simulink library "ddm"  (R2021b)
settings: Solver=VariableStepAuto  StartTime=0.0  StopTime=10.0  RelTol=1e-3
undefined symbols (not defined in the file or in its folder): ADDM_FrTMTqDev_X_Nm, ADDM_RrTMTqDev_X_Nm, ENUM_ADASACCSTA_ERROR, ENUM_ADASACCSTA_OFF, ENUM_ADASACCSTA_STANDBY, ENUM_ALLOWMOV_ALLOWREADY, ENUM_APS, ENUM_BRKSTA_ERROR, ENUM_BRKSTA_OFF, ENUM_BRKSTA_ON, ENUM_BRKSW_INVALID, ENUM_BRKSW_OFF, ENUM_BRKSW_ON, ENUM_CHGPREACTERRSTA_OBCPRE, ENUM_DCDCFAULTSTA_ANYFAULTLV1, ENUM_DCDCFAULTSTA_ANYFAULTLV2, ENUM_DRIVETRAIN_AWD, ENUM_DRIVETRAIN_FWD, ENUM_DRIVETRAIN_RWD, ENUM_EDUDRTSTA_NORMAL, ENUM_EPBSTA_APPLIED, ENUM_EPBSTA_RELEASED, ENUM_ESCAPSSta_APSUNAVAILABLE, ENUM_GEARACTUALPOSN_INVALID, ENUM_GEARACTUALPOSN_P, ENUM_HVBATTREADYPRE_READY, ENUM_MCUWARN_LV0, ENUM_MCUWARN_LV1, ENUM_MCUWARN_LV2, ENUM_MCUWARN_LV3, ENUM_MCUWARN_NOERROR, ENUM_OBCFAULTSTA_ANYFAULT, ENUM_PAS_R2F2, ENUM_PDFAULT_BATTPDFAIL, ENUM_PDFAULT_DCDCDISABLE, ENUM_PDFAULT_MCUDISABLE, ENUM_PDFAULT_MCUDISCHRG, ENUM_POWERSTA_OFF, ENUM_POWERSTA_ON, ENUM_POWERSTA_READY, ENUM_POWERSTA_STANDBY, ENUM_PRESSINDI_LOW, ENUM_PUFAULT_BATTUPFAIL, ENUM_PUFAULT_DCDCENABLEFAIL, ENUM_PUFAULT_PRECHRGCHKFAIL, ENUM_PUFAULT_SAFETYCHKFAIL, ENUM_PUSTATE_COMPLETED, ENUM_PWRSTASW_OFF, ENUM_PWRSTASW_OFFA, ENUM_PWRSTASW_OFFCHVCHRG, ENUM_PWRSTASW_OFFCLVCHRG, ENUM_PWRSTASW_ON, ENUM_PWRSTASW_ONHVCHRG, ENUM_PWRSTASW_READY, ENUM_PWRSTASW_STANDBY, ENUM_RAPSErrWarnSta_NORMAL, ENUM_RAPSErrWarnSta_RAPSERRLV1, ENUM_SHIFTCOMMAND_P, ENUM_SHIFTERERRSTA_PBUTTONFAILURE, ENUM_VEHMALFUNLV_2ND ... (+463)
libraries: hcu_lib x529, $bdroot x5, simulink x4
(part 19 of 25)

== system ddm/DDM/DDM/PMM/Fault level/Fault level 2 subsystem error ==
  note: Test Pass Criteria
  note: Release Condition After Failure Decision
  note: Diagnostics and Fault Handling
  note: Test Detection Criteria
  task_time_s : Inport
  VPMM_PowerSta_enum : Inport  Port=2
  VPMM_PwrStaSW_enum : Inport  Port=3
  VDDM_C3BMS6LCCFS_flg : Inport  Port=4
  VDDM_C3CCU2LCCFS_flg : Inport  Port=5
  VDDM_MCUNF1NoComCFS_flg : Inport  Port=6
  VDDM_MCUNR1NoComCFS_flg : Inport  Port=7
  VINP_BMSWarn4_flg : Inport  Port=8
  VINP_BMSWarn5_flg : Inport  Port=9
  VINP_DCDCFaultSta_enum : Inport  Port=10
  VINP_MCUWarnFNidec_enum : Inport  Port=11
  VINP_MCUWarnRNidec_enum : Inport  Port=12
  VPMM_DrivetrainSelect_enum : Inport  Port=13
  DTC_clear_request : Inport  Port=14
  No_CAN3_BUS_OFF : Inport  Port=15
  VDDM_C3CCU2RCCFS_flg : Inport  Port=16
  VDDM_C3CCU2CSCFS_flg : Inport  Port=17
  VDDM_MCUNR1RCErrCFS_flg : Inport  Port=18
  VDDM_MCUNR1CSErrCFS_flg : Inport  Port=19
  VDDM_MCUNF1RCErrCFS_flg : Inport  Port=20
  VDDM_MCUNF1CSErrCFS_flg : Inport  Port=21
  VDDM_C3BMS6RCCFS_flg : Inport  Port=22
  VDDM_C3BMS6CSCFS_flg : Inport  Port=23
  ZoneDrMalfunLevel_enum : Inport  Port=24
  No_CAN4_BUS_OFF : Inport  Port=25
  VDDM_DrVCUNoComCFS_flg : Inport  Port=26
  ZoneFrMalfunLevel_enum : Inport  Port=27
  VDDM_FrVCUNoComCFS_flg : Inport  Port=28
  AND1 : Logic  Inputs=5  AllPortsSameDT=off  OutDataTypeStr=boolean
  AND2 : Logic  Inputs=5  AllPortsSameDT=off  OutDataTypeStr=boolean
  AND5 : Logic  Inputs=3  AllPortsSameDT=off  OutDataTypeStr=boolean
  AND6 : Logic  Inputs=3  AllPortsSameDT=off  OutDataTypeStr=boolean
  Constant1 : Constant  Value=ENUM_PWRSTASW_OFF
  Constant14 : Constant  Value=ZERO_INT
  Constant15 : Constant  Value=KDDM_FaultLvDiagnosisOffSW_flg
  Constant16 : Constant  Value=ENUM_MCUWARN_LV1
  Constant17 : Constant  Value=ENUM_DRIVETRAIN_AWD
  Constant18 : Constant  Value=ENUM_DRIVETRAIN_AWD
  Constant19 : Constant  Value=KDDM_Lv2ErrPassTO_s
  Constant2 : Constant  Value=TRUE
  Constant20 : Constant  Value=ENUM_DRIVETRAIN_FWD
  Constant21 : Constant  Value=ENUM_DRIVETRAIN_RWD
  Constant22 : Constant  Value=ENUM_MCUWARN_LV2
  Constant23 : Constant  Value=ENUM_POWERSTA_OFF
  Constant24 : Constant  Value=TRUE
  Constant25 : Constant  Value=FALSE
  Constant26 : Constant  Value=ENUM_PWRSTASW_OFF
  Constant27 : Constant  Value=FALSE
  Constant28 : Constant  Value=ENUM_MCUWARN_LV1
  Constant3 : Constant  Value=KDDM_Lv2ErrDetTO_s
  Constant36 : Constant  Value=ENUM_DCDCFAULTSTA_ANYFAULTLV2
  Constant4 : Constant  Value=KDDM_Lv2ErrPassTO_s
  Constant40 : Constant  Value=KDDM_Lv2ErrDTC_cnt
  Constant5 : Constant  Value=KDDM_Lv2ErrDTC_cnt
  Constant6 : Constant  Value=ENUM_ZONEMALFUNLV_2ND
  Constant7 : Constant  Value=ENUM_ZONEMALFUNLV_2ND
  Constant8 : Constant  Value=FALSE
  Constant9 : Constant  Value=ENUM_MCUWARN_LV2
  DTC_Couter : hcu_lib/Basic_Blocks/DTC_Couter
  DTC_Info : hcu_lib/Basic_Blocks/DTC_Info
  Delay : Delay  DelayLength=1
  Equal : RelationalOperator  Operator=~=  OutDataTypeStr=boolean  RndMeth=Simplest
  Equal1 : RelationalOperator  Operator=~=  OutDataTypeStr=boolean  RndMeth=Simplest
  Equal{2,4..5,8,14,22..28} (12 alike) : RelationalOperator  Operator===  OutDataTypeStr=boolean  RndMeth=Simplest
  Equal3 : RelationalOperator  OutDataTypeStr=boolean  RndMeth=Simplest
  Logical Operator1 : Logic  Inputs=6  AllPortsSameDT=off  OutDataTypeStr=boolean
  Logical Operator2 : Logic  Inputs=6  AllPortsSameDT=off  OutDataTypeStr=boolean
  Logical Operator3 : Logic  AllPortsSameDT=off  OutDataTypeStr=boolean
  Logical Operator6 : Logic  Operator=NOT  AllPortsSameDT=off  OutDataTypeStr=boolean
  Logical Operator7 : Logic  Operator=OR  AllPortsSameDT=off  OutDataTypeStr=boolean
  Logical Operator8 : Logic  Operator=OR  Inputs=4  AllPortsSameDT=off  OutDataTypeStr=boolean
  Logical Operator9 : Logic  Operator=OR  AllPortsSameDT=off  OutDataTypeStr=boolean
  NOT{,5..7,9..13,15,17..19,26,28} (15 alike) : Logic  Operator=NOT  AllPortsSameDT=off  OutDataTypeStr=boolean
  OR : Logic  Operator=OR  AllPortsSameDT=off  OutDataTypeStr=boolean
  OR1 : Logic  Operator=OR  AllPortsSameDT=off  OutDataTypeStr=boolean
  OR2 : Logic  Operator=OR  Inputs=6  AllPortsSameDT=off  OutDataTypeStr=boolean
  OR3 : Logic  Operator=OR  Inputs=6  AllPortsSameDT=off  OutDataTypeStr=boolean
  OR4 : Logic  Operator=OR  AllPortsSameDT=off  OutDataTypeStr=boolean
  Relational Operator : RelationalOperator  Operator=>  OutDataTypeStr=boolean  RndMeth=Simplest
  Switch{1,4..5,9} (4 alike) : Switch  Criteria=u2 ~= 0
  Terminator : Terminator
  Test Detection Criteria : hcu_lib/Basic_Blocks/Test Detection Criteria
  Timer1 : hcu_lib/Basic_Blocks/Timer
  VDDM_Lv2ErrCFS_flg : Outport
  VDDM_Lv2ErrDTC_raw32 : Outport  Port=2
  wires:
  Constant9/1 -> Equal5/2
  [VINP_MCUWarnRNidec_enum] -> Equal5/1
  Equal5/1 -> OR4/2
  OR4/1 -> Logical Operator2/1
  Switch9/1 -> Test Detection Criteria/1
  Constant8/1 -> Switch9/1
  [VDDM_Lv2ErrCFSRls_flg] -> Switch9/2
  [VDDM_Lv2ErrCFS_flg] -> DTC_Info/3
  DTC_Info/1 -> VDDM_Lv2ErrDTC_raw32/1  "VDDM_Lv2ErrDTC_raw32"
  [VDDM_Lv2ErrPass_flg] -> DTC_Info/2
  [VDDM_Lv2ErrDet_flg] -> DTC_Info/1
  [DTC_clear_request] -> DTC_Info/4
  [VDDM_ZoneDrFaultLv2_flg] -> OR3/5
  [VDDM_ZoneFrFaultLv2_flg] -> OR3/6
  [VDDM_DCDCFaultLv2_flg] -> OR3/1
  [VDDM_BMSFaultLv2_flg] -> OR3/4
  [VDDM_MCUF1FaultLv2_flg] -> OR3/3
  [VDDM_MCUR1FaultLv2_flg] -> OR3/2
  VDDM_FrVCUNoComCFS_flg/1 -> [VDDM_FrVCUNoComCFS_flg]
  ZoneFrMalfunLevel_enum/1 -> [ZoneFrMalfunLevel_enum]
  VDDM_DrVCUNoComCFS_flg/1 -> [VDDM_DrVCUNoComCFS_flg]
  No_CAN4_BUS_OFF/1 -> [No_CAN4_BUS_OFF]
  ZoneDrMalfunLevel_enum/1 -> [ZoneDrMalfunLevel_enum]
  [VDDM_ZoneFrFaultLv2_flg] -> OR2/6
  [VDDM_ZoneDrFaultLv2_flg] -> OR2/5
  NOT28/1 -> AND6/3
  [VDDM_FrVCUNoComCFS_flg] -> NOT28/1
  Equal2/1 -> AND5/1
  Constant6/1 -> Equal2/2
  [VDDM_DrVCUNoComCFS_flg] -> NOT26/1
  AND5/1 -> [VDDM_ZoneDrFaultLv2_flg]  "VDDM_ZoneDrFaultLv2_flg"
  [No_CAN4_BUS_OFF] -> AND6/2
  AND6/1 -> [VDDM_ZoneFrFaultLv2_flg]  "VDDM_ZoneFrFaultLv2_flg"
  [ZoneDrMalfunLevel_enum] -> Equal2/1
  NOT26/1 -> AND5/3
  Equal8/1 -> AND6/1
  Constant7/1 -> Equal8/2
  [ZoneFrMalfunLevel_enum] -> Equal8/1
  [No_CAN4_BUS_OFF] -> AND5/2
  VDDM_C3BMS6CSCFS_flg/1 -> [VDDM_C3BMS6CSCFS_flg]
  VDDM_C3BMS6RCCFS_flg/1 -> [VDDM_C3BMS6RCCFS_flg]
  VDDM_MCUNF1CSErrCFS_flg/1 -> [VDDM_MCUNF1CSErrCFS_flg]
  VDDM_MCUNF1RCErrCFS_flg/1 -> [VDDM_MCUNF1RCErrCFS_flg]
  VDDM_MCUNR1CSErrCFS_flg/1 -> [VDDM_MCUNR1CSErrCFS_flg]
  VDDM_MCUNR1RCErrCFS_flg/1 -> [VDDM_MCUNR1RCErrCFS_flg]
  VDDM_C3CCU2CSCFS_flg/1 -> [VDDM_C3CCU2CSCFS_flg]
  VDDM_C3CCU2RCCFS_flg/1 -> [VDDM_C3CCU2RCCFS_flg]
  [VDDM_Lv2ErrCFS_flg] -> VDDM_Lv2ErrCFS_flg/1
  Constant1/1 -> Equal1/2
  Constant2/1 -> Switch1/3
  [VPMM_PwrStaSW_enum] -> Equal1/1
  Equal1/1 -> Switch1/2
  OR3/1 -> Switch1/1
  OR2/1 -> Switch5/1
  [VDDM_BMSFaultLv2_flg] -> OR2/4
  [VDDM_MCUF1FaultLv2_flg] -> OR2/3
  [VDDM_MCUR1FaultLv2_flg] -> OR2/2
  [VDDM_DCDCFaultLv2_flg] -> OR2/1
  NOT19/1 -> AND2/5
  [VDDM_C3BMS6CSCFS_flg] -> NOT19/1
  [VINP_BMSWarn4_flg] -> OR1/1
  [VINP_BMSWarn5_flg] -> OR1/2
  [VDDM_C3BMS6LCCFS_flg] -> NOT17/1
  NOT18/1 -> AND2/4
  [No_CAN3_BUS_OFF] -> AND2/2
  OR1/1 -> AND2/1
  [VDDM_C3BMS6RCCFS_flg] -> NOT18/1
  AND2/1 -> [VDDM_BMSFaultLv2_flg]  "VDDM_BMSFaultLv2_flg"
  NOT17/1 -> AND2/3
  OR/1 -> Logical Operator1/1
  Equal23/1 -> OR/2
  Equal28/1 -> OR/1
  Constant28/1 -> Equal28/2
  [VINP_MCUWarnFNidec_enum] -> Equal28/1
  Constant17/1 -> Equal27/2
  Equal25/1 -> Logical Operator7/1
  [VPMM_DrivetrainSelect_enum] -> Equal24/1, Equal22/2
  Constant21/1 -> Equal25/1
  [VINP_MCUWarnRNidec_enum] -> Equal26/1
  NOT9/1 -> Logical Operator2/3
  [VINP_MCUWarnFNidec_enum] -> Equal23/1
  Equal26/1 -> OR4/1
  NOT15/1 -> Logical Operator1/3
  NOT10/1 -> Logical Operator2/4
  [VDDM_MCUNR1RCErrCFS_flg] -> NOT10/1
  Logical Operator9/1 -> Logical Operator1/6
  [VDDM_MCUNF1CSErrCFS_flg] -> NOT13/1
  NOT12/1 -> Logical Operator1/4
  NOT13/1 -> Logical Operator1/5
  [VDDM_MCUNF1RCErrCFS_flg] -> NOT12/1
  [No_CAN3_BUS_OFF] -> Logical Operator1/2
  [VDDM_MCUNR1CSErrCFS_flg] -> NOT11/1
  Equal27/1 -> Logical Operator7/2
  Logical Operator1/1 -> [VDDM_MCUF1FaultLv2_flg]  "VDDM_MCUF1FaultLv2_flg"
  [No_CAN3_BUS_OFF] -> Logical Operator2/2
  Logical Operator2/1 -> [VDDM_MCUR1FaultLv2_flg]  "VDDM_MCUR1FaultLv2_flg"
  Constant16/1 -> Equal26/2
  [VDDM_MCUNR1NoComCFS_flg] -> NOT9/1
  Equal24/1 -> Logical Operator9/2
  NOT11/1 -> Logical Operator2/5
  Logical Operator7/1 -> Logical Operator2/6
  [VPMM_DrivetrainSelect_enum] -> Equal25/2, Equal27/1
  [VDDM_MCUF1NoComCFS_flg] -> NOT15/1
  Equal22/1 -> Logical Operator9/1
  Constant22/1 -> Equal23/2
  Constant18/1 -> Equal24/2
  Constant20/1 -> Equal22/1
  AND1/1 -> [VDDM_DCDCFaultLv2_flg]  "VDDM_DCDCFaultLv2_flg"
  [No_CAN3_BUS_OFF] -> AND1/2
  Equal14/1 -> AND1/1
  NOT6/1 -> AND1/4
  [VDDM_C3CCU2RCCFS_flg] -> NOT6/1
  NOT7/1 -> AND1/5
  [VDDM_C3CCU2CSCFS_flg] -> NOT7/1
  [VDDM_C3CCU2LCCFS_flg] -> NOT5/1
  NOT5/1 -> AND1/3
  Equal/1 -> Switch5/2
  Constant15/1 -> Logical Operator8/4
  [VDDM_Lv2ErrCFS_flg] -> Delay/1
  Delay/1 -> NOT/1
  NOT/1 -> Logical Operator3/2
  [VDDM_Lv2ErrPass_flg] -> Logical Operator3/1
  Logical Operator3/1 -> Logical Operator8/3
  [VDDM_Lv2ErrCFSRls_flg] -> DTC_Couter/2
  Constant14/1 -> Relational Operator/2
  Switch5/1 -> Switch9/3
  Constant3/1 -> Test Detection Criteria/4
  [task_time_s] -> Timer1/3
  No_CAN3_BUS_OFF/1 -> [No_CAN3_BUS_OFF]
  DTC_clear_request/1 -> [DTC_clear_request]
  [VPMM_PwrStaSW_enum] -> Equal/1
  [VPMM_PowerSta_enum] -> Equal4/1
  Constant4/1 -> Timer1/4
  Switch4/1 -> [VDDM_Lv2ErrCFSRls_flg]  "VDDM_Lv2ErrCFSRls_flg"
  [VINP_DCDCFaultSta_enum] -> Equal14/1
  Constant23/1 -> Equal4/2
  Constant25/1 -> Switch4/3
  Constant40/1 -> Test Detection Criteria/3
  DTC_Couter/2 -> Relational Operator/1  "VDDM_Lv2ErrDTC_cnt"
  DTC_Couter/1 -> [VDDM_Lv2ErrCFS_flg]  "VDDM_Lv2ErrCFS_flg"
  Equal4/1 -> Logical Operator8/1
  [DTC_clear_request] -> Logical Operator8/2
  Timer1/1 -> Equal3/1
  Relational Operator/1 -> Terminator/1  "VDDM_Lv2ErrDFS_flg"
  Constant19/1 -> Equal3/2
  [VDDM_Lv2ErrDet_flg] -> DTC_Couter/1
  Constant24/1 -> Switch4/1
  Switch1/1 -> Timer1/2, Logical Operator6/1
  Logical Operator8/1 -> Switch4/2
  Constant27/1 -> Switch5/3
  Constant26/1 -> Equal/2
  Constant36/1 -> Equal14/2
  Logical Operator6/1 -> Timer1/1
  [task_time_s] -> Test Detection Criteria/2
  Test Detection Criteria/1 -> [VDDM_Lv2ErrDet_flg]  "VDDM_Lv2ErrDet_flg"
  Equal3/1 -> [VDDM_Lv2ErrPass_flg]  "VDDM_Lv2ErrPass_flg"
  Constant5/1 -> DTC_Couter/3
  VDDM_C3BMS6LCCFS_flg/1 -> [VDDM_C3BMS6LCCFS_flg]
  VINP_BMSWarn4_flg/1 -> [VINP_BMSWarn4_flg]
  VINP_BMSWarn5_flg/1 -> [VINP_BMSWarn5_flg]
  task_time_s/1 -> [task_time_s]
  VPMM_PwrStaSW_enum/1 -> [VPMM_PwrStaSW_enum]
  VPMM_PowerSta_enum/1 -> [VPMM_PowerSta_enum]
  VDDM_C3CCU2LCCFS_flg/1 -> [VDDM_C3CCU2LCCFS_flg]
  VPMM_DrivetrainSelect_enum/1 -> [VPMM_DrivetrainSelect_enum]
  VINP_MCUWarnRNidec_enum/1 -> [VINP_MCUWarnRNidec_enum]
  VDDM_MCUNR1NoComCFS_flg/1 -> [VDDM_MCUNR1NoComCFS_flg]
  VDDM_MCUNF1NoComCFS_flg/1 -> [VDDM_MCUF1NoComCFS_flg]
  VINP_DCDCFaultSta_enum/1 -> [VINP_DCDCFaultSta_enum]
  VINP_MCUWarnFNidec_enum/1 -> [VINP_MCUWarnFNidec_enum]

== system ddm/DDM/DDM/PMM/Fault level/Fault level 3 subsystem error ==
  note: Release Condition After Failure Decision
  note: Diagnostics and Fault Handling
  note: Test Detection Criteria
  note: Test Pass Criteria
  task_time_s : Inport
  VPMM_PowerSta_enum : Inport  Port=2
  VPMM_PwrStaSW_enum : Inport  Port=3
  VDDM_C3BMS6LCCFS_flg : Inport  Port=4
  VDDM_MCUNF1NoComCFS_flg : Inport  Port=5
  VDDM_MCUNR1NoComCFS_flg : Inport  Port=6
  VINP_BMSWarn6_flg : Inport  Port=7
  VINP_MCUWarnFNidec_enum : Inport  Port=8
  VINP_MCUWarnRNidec_enum : Inport  Port=9
  VPMM_DrivetrainSelect_enum : Inport  Port=10
  DTC_clear_request : Inport  Port=11
  No_CAN3_BUS_OFF : Inport  Port=12
  VDDM_MCUNR1RCErrCFS_flg : Inport  Port=13
  VDDM_MCUNR1CSErrCFS_flg : Inport  Port=14
  VDDM_MCUNF1RCErrCFS_flg : Inport  Port=15
  VDDM_MCUNF1CSErrCFS_flg : Inport  Port=16
  VDDM_C3BMS6RCCFS_flg : Inport  Port=17
  VDDM_C3BMS6CSCFS_flg : Inport  Port=18
  ZoneDrMalfunLevel_enum : Inport  Port=19
  No_CAN4_BUS_OFF : Inport  Port=20
  VDDM_DrVCUNoComCFS_flg : Inport  Port=21
  ZoneFrMalfunLevel_enum : Inport  Port=22
  VDDM_FrVCUNoComCFS_flg : Inport  Port=23
  AND2 : Logic  Inputs=5  AllPortsSameDT=off  OutDataTypeStr=boolean
  AND5 : Logic  Inputs=3  AllPortsSameDT=off  OutDataTypeStr=boolean
  AND6 : Logic  Inputs=3  AllPortsSameDT=off  OutDataTypeStr=boolean
  Constant1 : Constant  Value=ENUM_PWRSTASW_OFF
  Constant10 : Constant  Value=ENUM_MCUWARN_LV3
  Constant11 : Constant  Value=ENUM_DRIVETRAIN_AWD
  Constant12 : Constant  Value=KDDM_FaultLvDiagnosisOffSW_flg
  Constant13 : Constant  Value=ENUM_DRIVETRAIN_RWD
  Constant14 : Constant  Value=ZERO_INT
  Constant15 : Constant  Value=ENUM_DRIVETRAIN_AWD
  Constant16 : Constant  Value=ENUM_DRIVETRAIN_FWD
  Constant17 : Constant  Value=ENUM_MCUWARN_LV3
  Constant18 : Constant  Value=KDDM_Lv3ErrPassTO_s
  Constant19 : Constant  Value=ENUM_POWERSTA_OFF
  Constant2 : Constant  Value=TRUE
  Constant20 : Constant  Value=ENUM_ZONEMALFUNLV_3RD
  Constant21 : Constant  Value=ENUM_ZONEMALFUNLV_3RD
  Constant22 : Constant  Value=FALSE
  Constant24 : Constant  Value=TRUE
  Constant25 : Constant  Value=FALSE
  Constant26 : Constant  Value=ENUM_PWRSTASW_OFF
  Constant27 : Constant  Value=FALSE
  Constant3 : Constant  Value=KDDM_Lv3ErrDetTO_s
  Constant4 : Constant  Value=KDDM_Lv3ErrPassTO_s
  Constant40 : Constant  Value=KDDM_Lv3ErrDTC_cnt
  Constant5 : Constant  Value=KDDM_Lv3ErrDTC_cnt
  DTC_Couter : hcu_lib/Basic_Blocks/DTC_Couter
  DTC_Info : hcu_lib/Basic_Blocks/DTC_Info
  Delay : Delay  DelayLength=1
  Equal : RelationalOperator  Operator=~=  OutDataTypeStr=boolean  RndMeth=Simplest
  Equal1 : RelationalOperator  Operator=~=  OutDataTypeStr=boolean  RndMeth=Simplest
  Equal{4,8..9,11..13,16..18} (9 alike) : RelationalOperator  Operator===  OutDataTypeStr=boolean  RndMeth=Simplest
  Equal3 : RelationalOperator  OutDataTypeStr=boolean  RndMeth=Simplest
  Logical Operator1 : Logic  Inputs=6  AllPortsSameDT=off  OutDataTypeStr=boolean
  Logical Operator2 : Logic  Operator=OR  AllPortsSameDT=off  OutDataTypeStr=boolean
  Logical Operator21 : Logic  AllPortsSameDT=off  OutDataTypeStr=boolean
  Logical Operator3 : Logic  Inputs=6  AllPortsSameDT=off  OutDataTypeStr=boolean
  Logical Operator6 : Logic  Operator=NOT  AllPortsSameDT=off  OutDataTypeStr=boolean
  Logical Operator8 : Logic  Operator=OR  Inputs=4  AllPortsSameDT=off  OutDataTypeStr=boolean
  Logical Operator9 : Logic  Operator=OR  AllPortsSameDT=off  OutDataTypeStr=boolean
  NOT{,9..13,15,17..19,26,28} (12 alike) : Logic  Operator=NOT  AllPortsSameDT=off  OutDataTypeStr=boolean
  OR : Logic  Operator=OR  Inputs=5  AllPortsSameDT=off  OutDataTypeStr=boolean
  OR1 : Logic  Operator=OR  Inputs=5  AllPortsSameDT=off  OutDataTypeStr=boolean
  Relational Operator : RelationalOperator  Operator=>  OutDataTypeStr=boolean  RndMeth=Simplest
  Switch{1,4..5,9} (4 alike) : Switch  Criteria=u2 ~= 0
  Terminator : Terminator
  Test Detection Criteria : hcu_lib/Basic_Blocks/Test Detection Criteria
  Timer1 : hcu_lib/Basic_Blocks/Timer
  VDDM_Lv3ErrCFS_flg : Outport
  VDDM_Lv3ErrDTC_raw32 : Outport  Port=2
  wires:
  Switch9/1 -> Test Detection Criteria/1
  Constant22/1 -> Switch9/1
  [VDDM_Lv3ErrCFSRls_flg] -> Switch9/2
  DTC_Info/1 -> VDDM_Lv3ErrDTC_raw32/1  "VDDM_Lv3ErrDTC_raw32"
  [VDDM_Lv3ErrCFS_flg] -> DTC_Info/3
  [VDDM_Lv3ErrPass_flg] -> DTC_Info/2
  [DTC_clear_request] -> DTC_Info/4
  [VDDM_Lv3ErrDet_flg] -> DTC_Info/1
  VDDM_FrVCUNoComCFS_flg/1 -> [VDDM_FrVCUNoComCFS_flg]
  ZoneFrMalfunLevel_enum/1 -> [ZoneFrMalfunLevel_enum]
  VDDM_DrVCUNoComCFS_flg/1 -> [VDDM_DrVCUNoComCFS_flg]
  No_CAN4_BUS_OFF/1 -> [No_CAN4_BUS_OFF]
  ZoneDrMalfunLevel_enum/1 -> [ZoneDrMalfunLevel_enum]
  VDDM_C3BMS6CSCFS_flg/1 -> [VDDM_C3BMS6CSCFS_flg]
  VDDM_C3BMS6RCCFS_flg/1 -> [VDDM_C3BMS6RCCFS_flg]
  VDDM_MCUNF1CSErrCFS_flg/1 -> [VDDM_MCUNF1CSErrCFS_flg]
  VDDM_MCUNF1RCErrCFS_flg/1 -> [VDDM_MCUNF1RCErrCFS_flg]
  VDDM_MCUNR1CSErrCFS_flg/1 -> [VDDM_MCUNR1CSErrCFS_flg]
  VDDM_MCUNR1RCErrCFS_flg/1 -> [VDDM_MCUNR1RCErrCFS_flg]
  [VDDM_Lv3ErrCFS_flg] -> VDDM_Lv3ErrCFS_flg/1
  OR1/1 -> Switch1/1
  [VDDM_ZoneFrFaultLv3_flg] -> OR1/5
  Constant2/1 -> Switch1/3
  Constant1/1 -> Equal1/2
  [VPMM_PwrStaSW_enum] -> Equal1/1
  [VDDM_ZoneDrFaultLv3_flg] -> OR1/4
  [VDDM_MCUF1FaultLv3_flg] -> OR1/2
  Equal1/1 -> Switch1/2
  [VDDM_BMSFaultLv3_flg] -> OR1/3
  [VDDM_MCUR1FaultLv3_flg] -> OR1/1
  OR/1 -> Switch5/1
  [VDDM_ZoneFrFaultLv3_flg] -> OR/5
  [VDDM_ZoneDrFaultLv3_flg] -> OR/4
  [VDDM_BMSFaultLv3_flg] -> OR/3
  [VDDM_MCUF1FaultLv3_flg] -> OR/2
  [VDDM_MCUR1FaultLv3_flg] -> OR/1
  Constant15/1 -> Equal13/2
  AND5/1 -> [VDDM_ZoneDrFaultLv3_flg]  "VDDM_ZoneDrFaultLv3_flg"
  [VDDM_C3BMS6CSCFS_flg] -> NOT19/1
  NOT19/1 -> AND2/5
  Constant21/1 -> Equal9/2
  NOT18/1 -> AND2/4
  [No_CAN4_BUS_OFF] -> AND5/2
  [ZoneFrMalfunLevel_enum] -> Equal9/1
  Equal9/1 -> AND6/1
  NOT26/1 -> AND5/3
  [ZoneDrMalfunLevel_enum] -> Equal8/1
  [VINP_BMSWarn6_flg] -> AND2/1
  [VDDM_DrVCUNoComCFS_flg] -> NOT26/1
  AND2/1 -> [VDDM_BMSFaultLv3_flg]  "VDDM_BMSFaultLv3_flg"
  NOT17/1 -> AND2/3
  Constant20/1 -> Equal8/2
  Equal8/1 -> AND5/1
  [No_CAN4_BUS_OFF] -> AND6/2
  AND6/1 -> [VDDM_ZoneFrFaultLv3_flg]  "VDDM_ZoneFrFaultLv3_flg"
  [VDDM_FrVCUNoComCFS_flg] -> NOT28/1
  NOT28/1 -> AND6/3
  [VDDM_C3BMS6RCCFS_flg] -> NOT18/1
  [No_CAN3_BUS_OFF] -> AND2/2
  [VDDM_C3BMS6LCCFS_flg] -> NOT17/1
  [VDDM_MCUNF1CSErrCFS_flg] -> NOT13/1
  Constant17/1 -> Equal12/2
  Equal13/1 -> Logical Operator9/2
  Constant16/1 -> Equal11/1
  [No_CAN3_BUS_OFF] -> Logical Operator3/2
  Logical Operator9/1 -> Logical Operator3/6
  [VDDM_MCUNF1NoComCFS_flg] -> NOT15/1
  NOT13/1 -> Logical Operator3/5
  NOT12/1 -> Logical Operator3/4
  Logical Operator3/1 -> [VDDM_MCUF1FaultLv3_flg]  "VDDM_MCUF1FaultLv3_flg"
  Equal11/1 -> Logical Operator9/1
  [VDDM_MCUNF1RCErrCFS_flg] -> NOT12/1
  [VPMM_DrivetrainSelect_enum] -> Equal13/1, Equal11/2
  [VINP_MCUWarnFNidec_enum] -> Equal12/1
  Equal12/1 -> Logical Operator3/1
  NOT15/1 -> Logical Operator3/3
  Equal17/1 -> Logical Operator1/1
  NOT9/1 -> Logical Operator1/3
  Equal18/1 -> Logical Operator2/2
  Equal16/1 -> Logical Operator2/1
  [VDDM_MCUNR1NoComCFS_flg] -> NOT9/1
  Constant11/1 -> Equal18/2
  Constant13/1 -> Equal16/1
  Constant10/1 -> Equal17/2
  [VINP_MCUWarnRNidec_enum] -> Equal17/1
  [VPMM_DrivetrainSelect_enum] -> Equal16/2, Equal18/1
  NOT10/1 -> Logical Operator1/4
  [No_CAN3_BUS_OFF] -> Logical Operator1/2
  [VDDM_MCUNR1CSErrCFS_flg] -> NOT11/1
  Logical Operator2/1 -> Logical Operator1/6
  Logical Operator1/1 -> [VDDM_MCUR1FaultLv3_flg]  "VDDM_MCUR1FaultLv3_flg"
  NOT11/1 -> Logical Operator1/5
  [VDDM_MCUNR1RCErrCFS_flg] -> NOT10/1
  Constant14/1 -> Relational Operator/2
  [VDDM_Lv3ErrCFSRls_flg] -> DTC_Couter/2
  Logical Operator21/1 -> Logical Operator8/3
  [VDDM_Lv3ErrCFS_flg] -> Delay/1
  NOT/1 -> Logical Operator21/2
  Delay/1 -> NOT/1
  Constant12/1 -> Logical Operator8/4
  [VDDM_Lv3ErrPass_flg] -> Logical Operator21/1
  Switch5/1 -> Switch9/3
  Constant3/1 -> Test Detection Criteria/4
  [task_time_s] -> Timer1/3
  No_CAN3_BUS_OFF/1 -> [No_CAN3_BUS_OFF]
  DTC_clear_request/1 -> [DTC_clear_request]
  [VPMM_PwrStaSW_enum] -> Equal/1
  [VPMM_PowerSta_enum] -> Equal4/1
  Constant4/1 -> Timer1/4
  Switch4/1 -> [VDDM_Lv3ErrCFSRls_flg]  "VDDM_Lv3ErrCFSRls_flg"
  Constant19/1 -> Equal4/2
  Constant25/1 -> Switch4/3
  Constant40/1 -> Test Detection Criteria/3
  DTC_Couter/2 -> Relational Operator/1  "VDDM_Lv3ErrDTC_cnt"
  DTC_Couter/1 -> [VDDM_Lv3ErrCFS_flg]  "VDDM_Lv3ErrCFS_flg"
  Equal4/1 -> Logical Operator8/1
  [DTC_clear_request] -> Logical Operator8/2
  Timer1/1 -> Equal3/1
  Constant26/1 -> Equal/2
  Relational Operator/1 -> Terminator/1  "VDDM_Lv3ErrDFS_flg"
  Constant18/1 -> Equal3/2
  Equal/1 -> Switch5/2
  [VDDM_Lv3ErrDet_flg] -> DTC_Couter/1
  Constant24/1 -> Switch4/1
  Switch1/1 -> Timer1/2, Logical Operator6/1
  Constant27/1 -> Switch5/3
  Logical Operator8/1 -> Switch4/2
  Logical Operator6/1 -> Timer1/1
  [task_time_s] -> Test Detection Criteria/2
  Test Detection Criteria/1 -> [VDDM_Lv3ErrDet_flg]  "VDDM_Lv3ErrDet_flg"
  Equal3/1 -> [VDDM_Lv3ErrPass_flg]  "VDDM_Lv3ErrPass_flg"
  Constant5/1 -> DTC_Couter/3
  VDDM_C3BMS6LCCFS_flg/1 -> [VDDM_C3BMS6LCCFS_flg]
  VINP_MCUWarnFNidec_enum/1 -> [VINP_MCUWarnFNidec_enum]
  VDDM_MCUNF1NoComCFS_flg/1 -> [VDDM_MCUNF1NoComCFS_flg]
  VDDM_MCUNR1NoComCFS_flg/1 -> [VDDM_MCUNR1NoComCFS_flg]
  VINP_MCUWarnRNidec_enum/1 -> [VINP_MCUWarnRNidec_enum]
  VPMM_DrivetrainSelect_enum/1 -> [VPMM_DrivetrainSelect_enum]
  VPMM_PowerSta_enum/1 -> [VPMM_PowerSta_enum]
  VPMM_PwrStaSW_enum/1 -> [VPMM_PwrStaSW_enum]
  task_time_s/1 -> [task_time_s]
  VINP_BMSWarn6_flg/1 -> [VINP_BMSWarn6_flg]

== system ddm/DDM/DDM/PMM/Fault level/Fault level 4 subsystem error1 ==
  note: Test Pass Criteria
  note: Release Condition After Failure Decision
  note: Diagnostics and Fault Handling
  note: Test Detection Criteria
  task_time_s : Inport
  VPMM_PowerSta_enum : Inport  Port=2
  VPMM_PwrStaSW_enum : Inport  Port=3
  VDDM_C3BMS6LCCFS_flg : Inport  Port=4
  VINP_BMSWarn7_flg : Inport  Port=5
  VINP_BMSWarn8_flg : Inport  Port=6
  DTC_clear_request : Inport  Port=7
  No_CAN3_BUS_OFF : Inport  Port=8
  VDDM_C3BMS6RCCFS_flg : Inport  Port=9
  VDDM_C3BMS6CSCFS_flg : Inport  Port=10
  ZoneDrMalfunLevel_enum : Inport  Port=11
  No_CAN4_BUS_OFF : Inport  Port=12
  VDDM_DrVCUNoComCFS_flg : Inport  Port=13
  ZoneFrMalfunLevel_enum : Inport  Port=14
  VDDM_FrVCUNoComCFS_flg : Inport  Port=15
  AND2 : Logic  Inputs=5  AllPortsSameDT=off  OutDataTypeStr=boolean
  AND5 : Logic  Inputs=3  AllPortsSameDT=off  OutDataTypeStr=boolean
  AND6 : Logic  Inputs=3  AllPortsSameDT=off  OutDataTypeStr=boolean
  Constant1 : Constant  Value=ENUM_PWRSTASW_OFF
  Constant12 : Constant  Value=KDDM_FaultLvDiagnosisOffSW_flg
  Constant14 : Constant  Value=ZERO_INT
  Constant18 : Constant  Value=KDDM_Lv4ErrPassTO_s
  Constant19 : Constant  Value=ENUM_POWERSTA_OFF
  Constant2 : Constant  Value=TRUE
  Constant22 : Constant  Value=FALSE
  Constant24 : Constant  Value=TRUE
  Constant25 : Constant  Value=FALSE
  Constant26 : Constant  Value=ENUM_PWRSTASW_OFF
  Constant27 : Constant  Value=FALSE
  Constant3 : Constant  Value=KDDM_Lv4ErrDetTO_s
  Constant4 : Constant  Value=KDDM_Lv4ErrPassTO_s
  Constant40 : Constant  Value=KDDM_Lv4ErrDTC_cnt
  Constant5 : Constant  Value=KDDM_Lv4ErrDTC_cnt
  Constant6 : Constant  Value=ENUM_ZONEMALFUNLV_4TH
  Constant7 : Constant  Value=ENUM_ZONEMALFUNLV_4TH
  DTC_Couter : hcu_lib/Basic_Blocks/DTC_Couter
  DTC_Info : hcu_lib/Basic_Blocks/DTC_Info
  Delay : Delay  DelayLength=1
  Equal : RelationalOperator  Operator=~=  OutDataTypeStr=boolean  RndMeth=Simplest
  Equal1 : RelationalOperator  Operator===  OutDataTypeStr=boolean  RndMeth=Simplest
  Equal2 : RelationalOperator  Operator=~=  OutDataTypeStr=boolean  RndMeth=Simplest
  Equal3 : RelationalOperator  OutDataTypeStr=boolean  RndMeth=Simplest
  Equal4 : RelationalOperator  Operator===  OutDataTypeStr=boolean  RndMeth=Simplest
  Equal8 : RelationalOperator  Operator===  OutDataTypeStr=boolean  RndMeth=Simplest
  Logical Operator21 : Logic  AllPortsSameDT=off  OutDataTypeStr=boolean
  Logical Operator6 : Logic  Operator=NOT  AllPortsSameDT=off  OutDataTypeStr=boolean
  Logical Operator8 : Logic  Operator=OR  Inputs=4  AllPortsSameDT=off  OutDataTypeStr=boolean
  NOT{,17..19,26,28} (6 alike) : Logic  Operator=NOT  AllPortsSameDT=off  OutDataTypeStr=boolean
  OR : Logic  Operator=OR  Inputs=3  AllPortsSameDT=off  OutDataTypeStr=boolean
  OR1 : Logic  Operator=OR  AllPortsSameDT=off  OutDataTypeStr=boolean
  OR2 : Logic  Operator=OR  Inputs=3  AllPortsSameDT=off  OutDataTypeStr=boolean
  Relational Operator : RelationalOperator  Operator=>  OutDataTypeStr=boolean  RndMeth=Simplest
  Switch{1,4..5,9} (4 alike) : Switch  Criteria=u2 ~= 0
  Terminator : Terminator
  Test Detection Criteria : hcu_lib/Basic_Blocks/Test Detection Criteria
  Timer1 : hcu_lib/Basic_Blocks/Timer
  VDDM_Lv4ErrCFS_flg : Outport
  VDDM_Lv4ErrDTC_raw32 : Outport  Port=2
  wires:
  Switch9/1 -> Test Detection Criteria/1
  Constant22/1 -> Switch9/1
  [VDDM_Lv4ErrCFSRls_flg] -> Switch9/2
  DTC_Info/1 -> VDDM_Lv4ErrDTC_raw32/1  "VDDM_Lv4ErrDTC_raw32"
  [VDDM_Lv4ErrPass_flg] -> DTC_Info/2
  [VDDM_Lv4ErrDet_flg] -> DTC_Info/1
  [VDDM_Lv4ErrCFS_flg] -> DTC_Info/3
  [DTC_clear_request] -> DTC_Info/4
  VDDM_FrVCUNoComCFS_flg/1 -> [VDDM_FrVCUNoComCFS_flg]
  ZoneFrMalfunLevel_enum/1 -> [ZoneFrMalfunLevel_enum]
  VDDM_DrVCUNoComCFS_flg/1 -> [VDDM_DrVCUNoComCFS_flg]
  No_CAN4_BUS_OFF/1 -> [No_CAN4_BUS_OFF]
  ZoneDrMalfunLevel_enum/1 -> [ZoneDrMalfunLevel_enum]
  VDDM_C3BMS6CSCFS_flg/1 -> [VDDM_C3BMS6CSCFS_flg]
  VDDM_C3BMS6RCCFS_flg/1 -> [VDDM_C3BMS6RCCFS_flg]
  [VDDM_Lv4ErrCFS_flg] -> VDDM_Lv4ErrCFS_flg/1
  Equal2/1 -> Switch1/2
  [VDDM_BMSFaultLv4_flg] -> OR2/1
  OR2/1 -> Switch1/1
  [VDDM_ZoneFrFaultLv4_flg] -> OR2/3
  Constant1/1 -> Equal2/2
  [VDDM_ZoneDrFaultLv4_flg] -> OR2/2
  [VPMM_PwrStaSW_enum] -> Equal2/1
  Constant2/1 -> Switch1/3
  OR/1 -> Switch5/1
  [VDDM_BMSFaultLv4_flg] -> OR/1
  [VDDM_ZoneDrFaultLv4_flg] -> OR/2
  [VDDM_ZoneFrFaultLv4_flg] -> OR/3
  AND5/1 -> [VDDM_ZoneDrFaultLv4_flg]  "VDDM_ZoneDrFaultLv4_flg"
  [VINP_BMSWarn7_flg] -> OR1/1
  [VDDM_C3BMS6CSCFS_flg] -> NOT19/1
  NOT19/1 -> AND2/5
  Constant7/1 -> Equal8/2
  NOT18/1 -> AND2/4
  [VINP_BMSWarn8_flg] -> OR1/2
  [No_CAN4_BUS_OFF] -> AND5/2
  [ZoneFrMalfunLevel_enum] -> Equal8/1
  Equal8/1 -> AND6/1
  NOT26/1 -> AND5/3
  [ZoneDrMalfunLevel_enum] -> Equal1/1
  OR1/1 -> AND2/1
  [VDDM_DrVCUNoComCFS_flg] -> NOT26/1
  AND2/1 -> [VDDM_BMSFaultLv4_flg]  "VDDM_BMSFaultLv4_flg"
  NOT17/1 -> AND2/3
  Constant6/1 -> Equal1/2
  Equal1/1 -> AND5/1
  [No_CAN4_BUS_OFF] -> AND6/2
  AND6/1 -> [VDDM_ZoneFrFaultLv4_flg]  "VDDM_ZoneFrFaultLv4_flg"
  [VDDM_FrVCUNoComCFS_flg] -> NOT28/1
  NOT28/1 -> AND6/3
  [VDDM_C3BMS6RCCFS_flg] -> NOT18/1
  [No_CAN3_BUS_OFF] -> AND2/2
  [VDDM_C3BMS6LCCFS_flg] -> NOT17/1
  Constant14/1 -> Relational Operator/2
  [VDDM_Lv4ErrCFSRls_flg] -> DTC_Couter/2
  [VDDM_Lv4ErrDet_flg] -> DTC_Couter/1
  [VDDM_Lv4ErrPass_flg] -> Logical Operator21/1
  Logical Operator21/1 -> Logical Operator8/3
  [VDDM_Lv4ErrCFS_flg] -> Delay/1
  Delay/1 -> NOT/1
  NOT/1 -> Logical Operator21/2
  Constant12/1 -> Logical Operator8/4
  Switch5/1 -> Switch9/3
  Constant3/1 -> Test Detection Criteria/4
  [task_time_s] -> Timer1/3
  No_CAN3_BUS_OFF/1 -> [No_CAN3_BUS_OFF]
  DTC_clear_request/1 -> [DTC_clear_request]
  [VPMM_PwrStaSW_enum] -> Equal/1
  [VPMM_PowerSta_enum] -> Equal4/1
  Constant4/1 -> Timer1/4
  Constant19/1 -> Equal4/2
  Constant25/1 -> Switch4/3
  Test Detection Criteria/1 -> [VDDM_Lv4ErrDet_flg]  "VDDM_Lv4ErrDet_flg"
  Constant27/1 -> Switch5/3
  Switch4/1 -> [VDDM_Lv4ErrCFSRls_flg]  "VDDM_Lv4ErrCFSRls_flg"
  Logical Operator8/1 -> Switch4/2
  Switch1/1 -> Timer1/2, Logical Operator6/1
  Equal/1 -> Switch5/2
  Constant24/1 -> Switch4/1
  Relational Operator/1 -> Terminator/1  "VDDM_Lv4ErrDFS_flg"
  DTC_Couter/1 -> [VDDM_Lv4ErrCFS_flg]  "VDDM_Lv4ErrCFS_flg"
  Constant18/1 -> Equal3/2
  Constant26/1 -> Equal/2
  Timer1/1 -> Equal3/1
  [DTC_clear_request] -> Logical Operator8/2
  Equal4/1 -> Logical Operator8/1
  Constant40/1 -> Test Detection Criteria/3
  DTC_Couter/2 -> Relational Operator/1  "VDDM_Lv4ErrDTC_cnt"
  [task_time_s] -> Test Detection Criteria/2
  Logical Operator6/1 -> Timer1/1
  Constant5/1 -> DTC_Couter/3
  Equal3/1 -> [VDDM_Lv4ErrPass_flg]  "VDDM_Lv4ErrPass_flg"
  VDDM_C3BMS6LCCFS_flg/1 -> [VDDM_C3BMS6LCCFS_flg]
  VINP_BMSWarn7_flg/1 -> [VINP_BMSWarn7_flg]
  task_time_s/1 -> [task_time_s]
  VPMM_PwrStaSW_enum/1 -> [VPMM_PwrStaSW_enum]
  VPMM_PowerSta_enum/1 -> [VPMM_PowerSta_enum]
  VINP_BMSWarn8_flg/1 -> [VINP_BMSWarn8_flg]

== system ddm/DDM/DDM/PMM/LV/Initial LV battery voltage too low ==
  note: Test Detection Criteria
  note: Test Pass Criteria
  note: Release Condition After Decision
  note: Diagnostics and Fault Handling
  task_time_s : Inport
  VPMM_PowerSta_enum : Inport  Port=2
  VPMM_PwrStaSW_enum : Inport  Port=3
  VINP_LVBattDet12V_V : Inport  Port=4
  VINP_CANMsgValidBMS5_flg : Inport  Port=5
  DTC_clear_request : Inport  Port=6
  Constant1 : Constant  Value=ENUM_PWRSTASW_OFF
  Constant12 : Constant  Value=ENUM_POWERSTA_STANDBY
  Constant13 : Constant  Value=ZERO_INT
  Constant17 : Constant  Value=KDDM_IniLVLoDTC_cnt
  Constant2 : Constant  Value=ENUM_PWRSTASW_OFF
  Constant22 : Constant  Value=KDDM_IniLVLoDetTO_s
  Constant23 : Constant  Value=FALSE
  Constant26 : Constant  Value=ENUM_PWRSTASW_STANDBY
  Constant27 : Constant  Value=FALSE
  Constant28 : Constant  Value=KDDM_IniLVLoPassTO_s
  Constant29 : Constant  Value=KDDM_IniLVLoPassTO_s
  Constant3 : Constant  Value=ENUM_PWRSTASW_STANDBY
  Constant30 : Constant  Value=KDDM_IniLVLoDTC_cnt
  Constant32 : Constant  Value=KDDM_LVDiagnosisOffSW_flg
  Constant33 : Constant  Value=ENUM_POWERSTA_OFF
  Constant34 : Constant  Value=KDDM_IniLVLoThd_mv
  Constant4 : Constant  Value=FALSE
  Constant5 : Constant  Value=KDDM_IniLVLoThd_mv
  DTC_Couter1 : hcu_lib/Basic_Blocks/DTC_Couter
  DTC_Info : hcu_lib/Basic_Blocks/DTC_Info
  Equal{1..2,4,11..12,14} (6 alike) : RelationalOperator  Operator===  OutDataTypeStr=boolean  RndMeth=Simplest
  Equal10 : RelationalOperator  OutDataTypeStr=boolean  RndMeth=Simplest
  Equal13 : RelationalOperator  Operator=<=  OutDataTypeStr=boolean  RndMeth=Simplest
  Equal3 : RelationalOperator  Operator=<=  OutDataTypeStr=boolean  RndMeth=Simplest
  Gain1 : Gain  Gain=1000
  Gain3 : Gain  Gain=1000
  Logical Operator : Logic  Operator=OR  AllPortsSameDT=off  OutDataTypeStr=boolean
  Logical Operator1 : Logic  Operator=OR  AllPortsSameDT=off  OutDataTypeStr=boolean
  Logical Operator14 : Logic  Operator=OR  Inputs=4  AllPortsSameDT=off  OutDataTypeStr=boolean
  Logical Operator16 : Logic  AllPortsSameDT=off  OutDataTypeStr=boolean
  Logical Operator17 : Logic  Operator=NOT  AllPortsSameDT=off  OutDataTypeStr=boolean
  Logical Operator2 : Logic  AllPortsSameDT=off  OutDataTypeStr=boolean
  Logical Operator9 : Logic  AllPortsSameDT=off  OutDataTypeStr=boolean
  Relational Operator1 : RelationalOperator  Operator=>  OutDataTypeStr=boolean  RndMeth=Simplest
  Switch1 : Switch  Criteria=u2 ~= 0
  Switch2 : Switch  Criteria=u2 ~= 0
  Switch7 : Switch  Criteria=u2 ~= 0
  Terminator : Terminator
  Test Detection Criteria1 : hcu_lib/Basic_Blocks/Test Detection Criteria
  Timer2 : hcu_lib/Basic_Blocks/Timer
  Unit Delay1 : UnitDelay  SampleTime=-1  HasFrameUpgradeWarning=on
  VDDM_IniLVLoDTC_raw32 : Outport
  VDDM_IniLVLoCFS_flg : Outport  Port=2
  wires:
  [VDDM_IniLVLoCFS_flg] -> VDDM_IniLVLoCFS_flg/1
  [VDDM_IniLVLoPass_flg] -> Logical Operator14/3
  Logical Operator9/1 -> Switch1/2
  Constant26/1 -> Equal14/1
  Equal13/1 -> Switch1/1
  Gain3/1 -> Equal13/1
  [VINP_LVBattDet12V_V] -> Gain3/1
  Constant34/1 -> Equal13/2
  DTC_Couter1/2 -> Relational Operator1/1  "VDDM_IniLVLoDTC_cnt"
  Constant28/1 -> Timer2/4
  DTC_Couter1/1 -> [VDDM_IniLVLoCFS_flg]  "VDDM_IniLVLoCFS_flg"
  [VDDM_IniLVLoDet_flg] -> DTC_Couter1/1
  Logical Operator16/1 -> Logical Operator14/1
  Unit Delay1/1 -> Equal11/1
  [DTC_clear_request] -> Logical Operator14/2
  Constant33/1 -> Equal11/2
  Equal11/1 -> Logical Operator16/1
  Test Detection Criteria1/1 -> [VDDM_IniLVLoDet_flg]  "VDDM_IniLVLoDet_flg"
  [VPMM_PowerSta_enum] -> Equal12/1
  Switch7/1 -> Test Detection Criteria1/1
  Constant32/1 -> Logical Operator14/4
  Constant12/1 -> Equal12/2
  [task_time_s] -> Timer2/3
  Logical Operator14/1 -> [VDDM_IniLVLoCFSRls_flg]  "VDDM_IniLVLoCFSRls_flg"
  Constant17/1 -> Test Detection Criteria1/3
  [VPMM_PowerSta_enum] -> Unit Delay1/1
  Relational Operator1/1 -> Terminator/1  "VDDM_IniLVLoDFS_flg"
  Equal12/1 -> Logical Operator16/2
  [task_time_s] -> Test Detection Criteria1/2
  Switch1/1 -> Switch7/3
  Constant30/1 -> DTC_Couter1/3
  Equal10/1 -> [VDDM_IniLVLoPass_flg]  "VDDM_IniLVLoPass_flg"
  [VDDM_IniLVLoCFSRls_flg] -> Switch7/2
  Constant23/1 -> Switch7/1
  Constant22/1 -> Test Detection Criteria1/4
  Constant29/1 -> Equal10/2
  Switch2/1 -> Logical Operator17/1, Timer2/2
  Timer2/1 -> Equal10/1
  Constant27/1 -> Switch1/3
  Logical Operator17/1 -> Timer2/1
  [VDDM_IniLVLoCFSRls_flg] -> DTC_Couter1/2
  Constant13/1 -> Relational Operator1/2
  task_time_s/1 -> [task_time_s]
  VINP_LVBattDet12V_V/1 -> [VINP_LVBattDet12V_V]
  VPMM_PwrStaSW_enum/1 -> [VPMM_PwrStaSW_enum]
  VPMM_PowerSta_enum/1 -> [VPMM_PowerSta_enum]
  DTC_clear_request/1 -> [DTC_clear_request]
  VINP_CANMsgValidBMS5_flg/1 -> [VINP_CANMsgValidBMS5_flg]
  DTC_Info/1 -> VDDM_IniLVLoDTC_raw32/1  "VDDM_IniLVLoDTC_raw32"
  [VDDM_IniLVLoPass_flg] -> DTC_Info/2
  [VDDM_IniLVLoCFS_flg] -> DTC_Info/3
  [VDDM_IniLVLoDet_flg] -> DTC_Info/1
  [DTC_clear_request] -> DTC_Info/4
  [VINP_CANMsgValidBMS5_flg] -> Logical Operator9/2
  Constant1/1 -> Equal1/2
  Constant5/1 -> Equal3/2
  Logical Operator2/1 -> Switch2/2
  [VINP_LVBattDet12V_V] -> Gain1/1
  Constant4/1 -> Switch2/3
  Equal3/1 -> Switch2/1
  Gain1/1 -> Equal3/1
  Logical Operator/1 -> Logical Operator9/1
  Equal14/1 -> Logical Operator/1
  Equal1/1 -> Logical Operator/2
  [VPMM_PwrStaSW_enum] -> Equal14/2, Equal1/1
  Equal4/1 -> Logical Operator1/1
  Constant2/1 -> Equal2/2
  Constant3/1 -> Equal4/1
  Logical Operator1/1 -> Logical Operator2/1
  [VPMM_PwrStaSW_enum] -> Equal4/2, Equal2/1
  Equal2/1 -> Logical Operator1/2
  [VINP_CANMsgValidBMS5_flg] -> Logical Operator2/2

== system ddm/DDM/DDM/PMM/LV/LV analog input error ==
  note: Diagnostics and Fault Handling
  note: Release Condition After Decision
  note: Test Pass Criteria
  note: Test Detection Criteria
  task_time_s : Inport
  VPMM_PowerSta_enum : Inport  Port=2
  VINP_LVBattDet12V_V : Inport  Port=3
  VINP_CANMsgValidBMS5_flg : Inport  Port=4
  DTC_clear_request : Inport  Port=5
  VDDM_AuxBattVolV_V : Inport  Port=6
  Abs : Abs
  Abs1 : Abs
  Add : Sum  Inputs=-+
  Add1 : Sum  Inputs=-+
  Constant : Constant  Value=eps
  Constant1 : Constant  Value=eps
  Constant12 : Constant  Value=ENUM_POWERSTA_STANDBY
  Constant13 : Constant  Value=ZERO_INT
  Constant17 : Constant  Value=KDDM_LVInErrDTC_cnt
  Constant2 : Constant  Value=FALSE
  Constant22 : Constant  Value=KDDM_LVInErrDetTO_s
  Constant23 : Constant  Value=FALSE
  Constant27 : Constant  Value=FALSE
  Constant28 : Constant  Value=KDDM_LVInErrPassTO_s
  Constant3 : Constant  Value=KDDM_LVInErr_pct
  Constant30 : Constant  Value=KDDM_LVInErrDTC_cnt
  Constant32 : Constant  Value=KDDM_LVDiagnosisOffSW_flg
  Constant33 : Constant  Value=ENUM_POWERSTA_OFF
  Constant34 : Constant  Value=KDDM_LVInErr_pct
  Constant4 : Constant  Value=KDDM_LVInErrPassTO_s
  DTC_Couter1 : hcu_lib/Basic_Blocks/DTC_Couter
  DTC_Info : hcu_lib/Basic_Blocks/DTC_Info
  Divide : Product  Inputs=*/
  Divide1 : Product  Inputs=*/
  Equal1 : RelationalOperator  OutDataTypeStr=boolean  RndMeth=Simplest
  Equal10 : RelationalOperator  OutDataTypeStr=boolean  RndMeth=Simplest
  Equal11 : RelationalOperator  Operator===  OutDataTypeStr=boolean  RndMeth=Simplest
  Equal12 : RelationalOperator  Operator===  OutDataTypeStr=boolean  RndMeth=Simplest
  Equal13 : RelationalOperator  OutDataTypeStr=boolean  RndMeth=Simplest
  Gain : Gain  Gain=100  OutDataTypeStr=single
  Gain1 : Gain  Gain=100  OutDataTypeStr=single
  Logical Operator14 : Logic  Operator=OR  Inputs=4  AllPortsSameDT=off  OutDataTypeStr=boolean
  Logical Operator16 : Logic  AllPortsSameDT=off  OutDataTypeStr=boolean
  Logical Operator17 : Logic  Operator=NOT  AllPortsSameDT=off  OutDataTypeStr=boolean
  Max : MinMax  Function=max  Inputs=2
  Max1 : MinMax  Function=max  Inputs=2
  Relational Operator1 : RelationalOperator  Operator=>  OutDataTypeStr=boolean  RndMeth=Simplest
  Switch1 : Switch  Criteria=u2 ~= 0
  Switch2 : Switch  Criteria=u2 ~= 0
  Switch7 : Switch  Criteria=u2 ~= 0
  Terminator : Terminator
  Test Detection Criteria1 : hcu_lib/Basic_Blocks/Test Detection Criteria
  Timer2 : hcu_lib/Basic_Blocks/Timer
  Unit Delay1 : UnitDelay  SampleTime=-1  HasFrameUpgradeWarning=on
  VDDM_LVInErrDTC_raw32 : Outport
  VDDM_LVInErrCFS_flg : Outport  Port=2
  wires:
  [VDDM_LVInErrCFS_flg] -> VDDM_LVInErrCFS_flg/1
  Constant2/1 -> Switch2/3
  [VDDM_AuxBattVolV_V] -> Add1/1
  [VINP_CANMsgValidBMS5_flg] -> Switch2/2
  Constant3/1 -> Equal1/2
  Equal1/1 -> Switch2/1
  [VINP_LVBattDet12V_V] -> Add1/2, Max1/1
  Gain1/1 -> Equal1/1
  Add1/1 -> Divide1/1
  Divide1/1 -> Abs1/1
  Abs1/1 -> Gain1/1
  Constant1/1 -> Max1/2
  Max1/1 -> Divide1/2
  Max/1 -> Divide/2
  Add/1 -> Divide/1
  Constant/1 -> Max/2
  [VINP_LVBattDet12V_V] -> Add/2, Max/1
  [VDDM_AuxBattVolV_V] -> Add/1
  Abs/1 -> Gain/1
  Divide/1 -> Abs/1
  VDDM_AuxBattVolV_V/1 -> [VDDM_AuxBattVolV_V]
  VPMM_PowerSta_enum/1 -> [VPMM_PowerSta_enum]
  VINP_LVBattDet12V_V/1 -> [VINP_LVBattDet12V_V]
  VINP_CANMsgValidBMS5_flg/1 -> [VINP_CANMsgValidBMS5_flg]
  [DTC_clear_request] -> DTC_Info/4
  DTC_clear_request/1 -> [DTC_clear_request]
  [VDDM_LVInErrCFS_flg] -> DTC_Info/3
  task_time_s/1 -> [task_time_s]
  DTC_Info/1 -> VDDM_LVInErrDTC_raw32/1  "VDDM_LVInErrDTC_raw32"
  [VDDM_LVInErrDet_flg] -> DTC_Info/1
  [VDDM_LVInErrPass_flg] -> DTC_Info/2
  Equal10/1 -> [VDDM_LVInErrPass_flg]  "VDDM_LVInErrPass_flg"
  Constant23/1 -> Switch7/1
  Constant13/1 -> Relational Operator1/2
  [VDDM_LVInErrCFSRls_flg] -> Switch7/2
  Constant34/1 -> Equal13/2
  DTC_Couter1/1 -> [VDDM_LVInErrCFS_flg]  "VDDM_LVInErrCFS_flg"
  Equal12/1 -> Logical Operator16/2
  [VDDM_LVInErrCFSRls_flg] -> DTC_Couter1/2
  [VPMM_PowerSta_enum] -> Equal12/1
  Constant12/1 -> Equal12/2
  Switch7/1 -> Test Detection Criteria1/1
  Gain/1 -> Equal13/1
  Constant33/1 -> Equal11/2
  [task_time_s] -> Timer2/3
  Constant30/1 -> DTC_Couter1/3
  Relational Operator1/1 -> Terminator/1  "VDDM_LVInErrDFS_flg"
  Constant22/1 -> Test Detection Criteria1/4
  Logical Operator14/1 -> [VDDM_LVInErrCFSRls_flg]  "VDDM_LVInErrCFSRls_flg"
  Constant27/1 -> Switch1/3
  [VDDM_LVInErrPass_flg] -> Logical Operator14/3
  [VPMM_PowerSta_enum] -> Unit Delay1/1
  Constant17/1 -> Test Detection Criteria1/3
  Unit Delay1/1 -> Equal11/1
  Constant4/1 -> Equal10/2
  Equal11/1 -> Logical Operator16/1
  [VINP_CANMsgValidBMS5_flg] -> Switch1/2
  [DTC_clear_request] -> Logical Operator14/2
  Equal13/1 -> Switch1/1
  [VDDM_LVInErrDet_flg] -> DTC_Couter1/1
  Logical Operator17/1 -> Timer2/1
  DTC_Couter1/2 -> Relational Operator1/1  "VDDM_LVInErrDTC_cnt"
  Logical Operator16/1 -> Logical Operator14/1
  Timer2/1 -> Equal10/1
  Test Detection Criteria1/1 -> [VDDM_LVInErrDet_flg]  "VDDM_LVInErrDet_flg"
  Switch1/1 -> Switch7/3
  Constant28/1 -> Timer2/4
  Switch2/1 -> Logical Operator17/1, Timer2/2
  Constant32/1 -> Logical Operator14/4
  [task_time_s] -> Test Detection Criteria1/2

== system ddm/DDM/DDM/PMM/LV/LV power supply voltage too high ==
  note: Release Condition After Decision
  note: Test Detection Criteria
  note: Test Pass Criteria
  note: Diagnostics and Fault Handling
  task_time_s : Inport
  VPMM_PowerSta_enum : Inport  Port=2
  VPMM_PwrStaSW_enum : Inport  Port=3
  VINP_LVBattDet12V_V : Inport  Port=4
  VINP_CANMsgValidBMS5_flg : Inport  Port=5
  DTC_clear_request : Inport  Port=6
  Constant28 : Constant  Value=ENUM_POWERSTA_STANDBY
  Constant29 : Constant  Value=ZERO_INT
  Constant30 : Constant  Value=KDDM_LVSupHiDTC_cnt
  Constant31 : Constant  Value=KDDM_LVSupHiDetTO_s
  Constant32 : Constant  Value=KDDM_LVSupHiPassTO_s
  Constant33 : Constant  Value=FALSE
  Constant34 : Constant  Value=ENUM_PWRSTASW_READY
  Constant35 : Constant  Value=ENUM_PWRSTASW_OFFCHVCHRG
  Constant36 : Constant  Value=ENUM_PWRSTASW_READY
  Constant37 : Constant  Value=ENUM_PWRSTASW_OFFCHVCHRG
  Constant38 : Constant  Value=ENUM_PWRSTASW_ON
  Constant39 : Constant  Value=ENUM_PWRSTASW_OFFCLVCHRG
  Constant42 : Constant  Value=KDDM_LVDiagnosisOffSW_flg
  Constant43 : Constant  Value=ENUM_POWERSTA_OFF
  Constant44 : Constant  Value=ENUM_PWRSTASW_ON
  Constant45 : Constant  Value=ENUM_PWRSTASW_ONHVCHRG
  Constant47 : Constant  Value=ENUM_PWRSTASW_OFFCLVCHRG
  Constant49 : Constant  Value=ENUM_PWRSTASW_ONHVCHRG
  Constant50 : Constant  Value=FALSE
  Constant51 : Constant  Value=KDDM_LVSupHiThd_mv
  Constant52 : Constant  Value=ENUM_PWRSTASW_OFFA
  Constant53 : Constant  Value=FALSE
  Constant54 : Constant  Value=KDDM_LVSupHiThd_mv
  Constant55 : Constant  Value=ENUM_PWRSTASW_OFFA
  Constant56 : Constant  Value=KDDM_LVSupHiPassTO_s
  Constant57 : Constant  Value=KDDM_LVSupHiDTC_cnt
  DTC_Couter1 : hcu_lib/Basic_Blocks/DTC_Couter
  DTC_Info : hcu_lib/Basic_Blocks/DTC_Info
  Delay1 : Delay  DelayLength=1
  Equal16 : RelationalOperator  OutDataTypeStr=boolean  RndMeth=Simplest
  Equal{17..24,26..29,31..32} (14 alike) : RelationalOperator  Operator===  OutDataTypeStr=boolean  RndMeth=Simplest
  Equal25 : RelationalOperator  OutDataTypeStr=boolean  RndMeth=Simplest
  Equal30 : RelationalOperator  OutDataTypeStr=boolean  RndMeth=Simplest
  Gain3 : Gain  Gain=KXX2XX
  Gain4 : Gain  Gain=KXX2XX
  Logical Operator{9..11,16} (4 alike) : Logic  AllPortsSameDT=off  OutDataTypeStr=boolean
  Logical Operator14 : Logic  Operator=OR  Inputs=4  AllPortsSameDT=off  OutDataTypeStr=boolean
  Logical Operator17 : Logic  Operator=NOT  AllPortsSameDT=off  OutDataTypeStr=boolean
  NOT1 : Logic  Operator=NOT  AllPortsSameDT=off  OutDataTypeStr=boolean
  OR2 : Logic  Operator=OR  Inputs=6  AllPortsSameDT=off  OutDataTypeStr=boolean
  OR3 : Logic  Operator=OR  Inputs=6  AllPortsSameDT=off  OutDataTypeStr=boolean
  Relational Operator1 : RelationalOperator  Operator=>  OutDataTypeStr=boolean  RndMeth=Simplest
  Switch1 : Switch  Criteria=u2 ~= 0
  Switch5 : Switch  Criteria=u2 ~= 0
  Switch7 : Switch  Criteria=u2 ~= 0
  Terminator : Terminator
  Test Detection Criteria1 : hcu_lib/Basic_Blocks/Test Detection Criteria
  Timer2 : hcu_lib/Basic_Blocks/Timer
  Unit Delay1 : UnitDelay  SampleTime=-1  HasFrameUpgradeWarning=on
  VDDM_LVSupHiDTC_raw32 : Outport
  VDDM_LVSupHiCFS_flg : Outport  Port=2
  wires:
  [VDDM_LVSupHiCFS_flg] -> VDDM_LVSupHiCFS_flg/1
  [VINP_LVBattDet12V_V] -> Gain4/1
  Gain4/1 -> Equal30/1
  Constant54/1 -> Equal30/2
  Constant51/1 -> Equal25/2
  Gain3/1 -> Equal25/1
  [VINP_LVBattDet12V_V] -> Gain3/1
  [VINP_CANMsgValidBMS5_flg] -> Logical Operator10/2
  Equal17/1 -> Logical Operator16/1
  Equal18/1 -> Logical Operator16/2
  Unit Delay1/1 -> Equal17/1
  DTC_Couter1/1 -> [VDDM_LVSupHiCFS_flg]  "VDDM_LVSupHiCFS_flg"
  Constant28/1 -> Equal18/2
  Equal22/1 -> OR3/1
  [VPMM_PowerSta_enum] -> Equal18/1
  Constant42/1 -> Logical Operator14/4
  [task_time_s] -> Timer2/3
  [VINP_CANMsgValidBMS5_flg] -> Logical Operator9/2
  [task_time_s] -> Test Detection Criteria1/2
  Equal16/1 -> [VDDM_LVSupHiPass_flg]  "VDDM_LVSupHiPass_flg"
  [VPMM_PowerSta_enum] -> Unit Delay1/1
  [VPMM_PwrStaSW_enum] -> Equal23/2, Equal24/1
  Constant33/1 -> Switch7/1
  Constant29/1 -> Relational Operator1/2
  DTC_Couter1/2 -> Relational Operator1/1  "VDDM_LVSupHiDTC_cnt"
  Logical Operator17/1 -> Timer2/1
  Constant45/1 -> Equal21/2
  Timer2/1 -> Equal16/1
  Equal27/1 -> OR2/3
  Logical Operator16/1 -> Logical Operator14/1
  Constant43/1 -> Equal17/2
  Switch7/1 -> Test Detection Criteria1/1
  [DTC_clear_request] -> Logical Operator14/2
  [VPMM_PwrStaSW_enum] -> Equal22/2, Equal21/1
  Logical Operator10/1 -> Switch5/2
  Constant38/1 -> Equal22/1
  Constant55/1 -> Equal31/2
  Equal26/1 -> OR2/4
  [VPMM_PwrStaSW_enum] -> Equal32/2, Equal31/1
  Constant53/1 -> Switch5/3
  Equal30/1 -> Switch5/1
  OR3/1 -> Logical Operator10/1
  Equal28/1 -> OR3/5
  Equal32/1 -> OR3/3
  Constant37/1 -> Equal28/1
  Constant36/1 -> Equal32/1
  Equal24/1 -> OR2/6
  Constant39/1 -> Equal29/2
  [VPMM_PwrStaSW_enum] -> Equal28/2, Equal29/1
  Equal29/1 -> OR3/6
  Equal21/1 -> OR3/2
  Equal31/1 -> OR3/4
  Constant30/1 -> Test Detection Criteria1/3
  Constant31/1 -> Test Detection Criteria1/4
  Logical Operator11/1 -> Logical Operator14/3
  OR2/1 -> Logical Operator9/1
  Constant35/1 -> Equal23/1
  Constant47/1 -> Equal24/2
  Equal19/1 -> OR2/2
  Constant44/1 -> Equal20/1
  Constant34/1 -> Equal27/1
  Equal23/1 -> OR2/5
  Equal25/1 -> Switch1/1
  Constant52/1 -> Equal26/2
  [VPMM_PwrStaSW_enum] -> Equal27/2, Equal26/1
  Equal20/1 -> OR2/1
  Constant49/1 -> Equal19/2
  Constant50/1 -> Switch1/3
  Logical Operator9/1 -> Switch1/2
  [VPMM_PwrStaSW_enum] -> Equal20/2, Equal19/1
  [VDDM_LVSupHiCFS_flg] -> Delay1/1
  [VDDM_LVSupHiCFSRls_flg] -> DTC_Couter1/2
  [VDDM_LVSupHiPass_flg] -> Logical Operator11/1
  [VDDM_LVSupHiDet_flg] -> DTC_Couter1/1
  Constant57/1 -> DTC_Couter1/3
  NOT1/1 -> Logical Operator11/2
  Delay1/1 -> NOT1/1
  Test Detection Criteria1/1 -> [VDDM_LVSupHiDet_flg]  "VDDM_LVSupHiDet_flg"
  Logical Operator14/1 -> [VDDM_LVSupHiCFSRls_flg]  "VDDM_LVSupHiCFSRls_flg"
  [VDDM_LVSupHiCFSRls_flg] -> Switch7/2
  Constant56/1 -> Equal16/2
  Relational Operator1/1 -> Terminator/1  "VDDM_LVSupHiDFS_flg"
  Constant32/1 -> Timer2/4
  Switch5/1 -> Timer2/2, Logical Operator17/1
  Switch1/1 -> Switch7/3
  task_time_s/1 -> [task_time_s]
  VINP_LVBattDet12V_V/1 -> [VINP_LVBattDet12V_V]
  DTC_clear_request/1 -> [DTC_clear_request]
  VINP_CANMsgValidBMS5_flg/1 -> [VINP_CANMsgValidBMS5_flg]
  VPMM_PowerSta_enum/1 -> [VPMM_PowerSta_enum]
  VPMM_PwrStaSW_enum/1 -> [VPMM_PwrStaSW_enum]
  DTC_Info/1 -> VDDM_LVSupHiDTC_raw32/1  "VDDM_LVSupHiDTC_raw32"
  [VDDM_LVSupHiPass_flg] -> DTC_Info/2
  [VDDM_LVSupHiCFS_flg] -> DTC_Info/3
  [VDDM_LVSupHiDet_flg] -> DTC_Info/1
  [DTC_clear_request] -> DTC_Info/4
